simulink model "snake"  (R2018a)
settings: Solver=VariableStepAuto  StartTime=0.0  StopTime=10.0  RelTol=1e-3
settings Model: Creator=12037  LastModifiedBy=12037

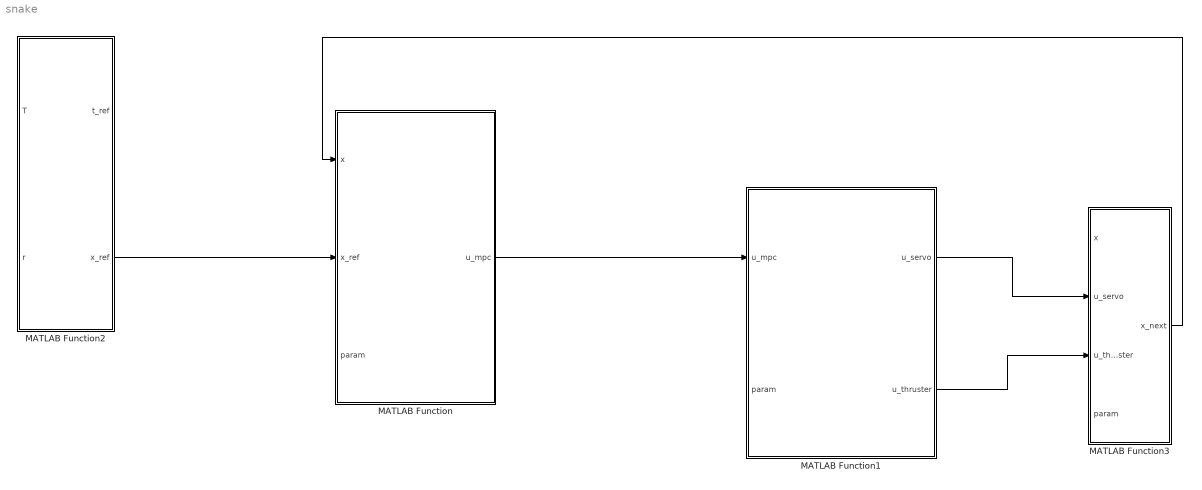
== system snake ==
  MATLAB Function : MATLAB Function  TreatAsAtomicUnit=on
  MATLAB Function1 : MATLAB Function  TreatAsAtomicUnit=on
  MATLAB Function2 : MATLAB Function  TreatAsAtomicUnit=on
  MATLAB Function3 : MATLAB Function  TreatAsAtomicUnit=on
  wires:
  MATLAB Function/1(u_mpc) -> MATLAB Function1/1(u_mpc)
  MATLAB Function2/2(x_ref) -> MATLAB Function/2(x_ref)
  MATLAB Function1/1(u_servo) -> MATLAB Function3/2(u_servo)
  MATLAB Function1/2(u_thruster) -> MATLAB Function3/3(u_thruster)
  MATLAB Function3/1(x_next) -> MATLAB Function/1(x)

== matlab function snake/MATLAB Function1 ==
  data: u_mpc input; u_servo output; param input; u_thruster output
% 基于优先级的全身控制（8舵机+8推进器）
function [u_servo, u_thruster] = wbc_allocator(u_mpc, param)
    %% 1. 任务雅可比（根据机械结构计算）
    J_servo = get_servo_jacobian();  % 舵机运动学雅可比 (3x8)
    J_thruster = get_thruster_jacobian(); % 推进器雅可比 (3x8)
    
    %% 2. 优先级分配（姿态>力控制>冗余优化）
    J = [J_servo; J_thruster]; % 6x16
    H = J'*J + 1e-3*eye(16);  % 正则化防止奇异性
    f = -J'*u_mpc;
    
    %% 3. 执行器约束
    u_servo_lim = param.u_servo_max*ones(8,1);
    u_thruster_lim = param.u_thruster_max*ones(8,1);
    A = eye(16);
    lb = [-u_servo_lim; -u_thruster_lim];
    ub = [ u_servo_lim;  u_thruster_lim];
    
    %% 4. 求解（使用quadprog）
    options = optimoptions('quadprog','Display','off');
    u = quadprog(H, f, A, [], [], [], lb, ub, [], options);
    
    u_servo = u(1:8);    % 舵机输出（力矩）
    u_thruster = u(9:16);% 推进器输出（推力）
end

== matlab function snake/MATLAB Function ==
  data: x input; u_mpc output; x_ref input; param input
% 带约束的非线性MPC（姿态优先）
function u_mpc = mpc_controller(x, x_ref, param)
    %% 1. 动力学建模（离散化）
    A = eye(13) + param.dt*[
        zeros(3), eye(3), zeros(3), zeros(3,1);  % 姿态运动学
        zeros(3), zeros(3), eye(3), zeros(3,1);  % 位置积分
        zeros(3), zeros(3), -param.D/param.m, zeros(3,1); % 速度动力学
        zeros(1,12), 1                           % 重力补偿
    ];
    B = param.dt*[
        zeros(6,15);                          % 姿态/位置无直接控制
        inv(param.I)*compute_force_jacobian(); % 力矩雅可比（需根据连杆结构计算）
        eye(3)/param.m                        % 线加速度
    ];
    
    %% 2. 代价函数（姿态误差权重最高）
    e_pos = x(4:6) - x_ref(4:6);
    e_ori = x(1:3) - x_ref(1:3); % 欧拉角误差
    J = e_pos'*param.Q(4:6,4:6)*e_pos + 100*e_ori'*param.Q(1:3,1:3)*e_ori;
    
    %% 3. 约束处理（接触力限制）
    u_min = -param.u_thruster_max*ones(15,1);
    u_max = param.u_thruster_max*ones(15,1);
    
    %% 4. 求解（使用QP简化版）
    H = 2*param.R;
    g = 2*param.R*(u_min + u_max)/2; % 趋向中间值
    u_mpc = quadprog(H, g, [], [], [], [], u_min, u_max);
end

== matlab function snake/MATLAB Function2 ==
  data: T input; t_ref output; r input; x_ref output
% 海底管道蛇形轨迹生成（带姿态对准）
function [t_ref, x_ref] = generate_pipe_trajectory(T, r)
    t = 0:0.05:T;
    N = length(t);
    
    % 螺旋上升轨迹（模拟管道弯曲）
    x_ref = zeros(13, N);
    x_ref(4,:) = 0.5*t;          % 沿管道轴向移动 (m)
    x_ref(6,:) = r*cos(2*pi*t/10); % 管道截面y坐标
    x_ref(5,:) = r*sin(2*pi*t/10); % 管道截面z坐标
    
    % 姿态对准管道方向（偏航角跟随管道曲率）
    x_ref(3,:) = atan2(diff(x_ref(5,:)), diff(x_ref(4,:))); 
    x_ref(3,1) = 0; % 初始偏航角
    
    % 参考速度（根据任务调整）
    x_ref(10,:) = 0.5; % 轴向速度
    
    t_ref = t';
end

== matlab function snake/MATLAB Function3 ==
  data: x input; x_next output; u_servo input; u_thruster input; param input
% 带流体动力学的刚体模型（反馈闭环）
function x_next = robot_dynamics(x, u_servo, u_thruster, param)
    %% 1. 姿态动力学（欧拉角形式）
    [roll, pitch, yaw] = x(1:3);
    R = Rotz(yaw)*Roty(pitch)*Rotx(roll); % 旋转矩阵
    
    %% 2. 线速度与角速度
    v_body = x(10:12);         % 体坐标系速度
    omega = x(7:9);            % 角速度
    
    %% 3. 合力与力矩（含推进器和舵机）
    F_total = sum(u_thruster) - param.D*v_body; % 水阻力
    tau_total = u_servo;       % 舵机提供的力矩
    
    %% 4. 状态更新（离散积分）
    dx = [
        omega;                  % 欧拉角速率（需运动学转换）
        R*v_body;               % 世界坐标系位置变化
        inv(param.I)*(tau_total - cross(omega, param.I*omega)); % 角速度微分
        F_total/param.m;        % 线加速度
        0                       % 重力/浮力平衡
    ];
    
    x_next = x + param.dt*dx;
end
